simulink model "prob1"  (R2020b)
settings: Solver=VariableStepAuto  StartTime=0.0  StopTime=10.0  RelTol=1e-3
settings Model: Creator=Nitin  LastModifiedBy=Nitin

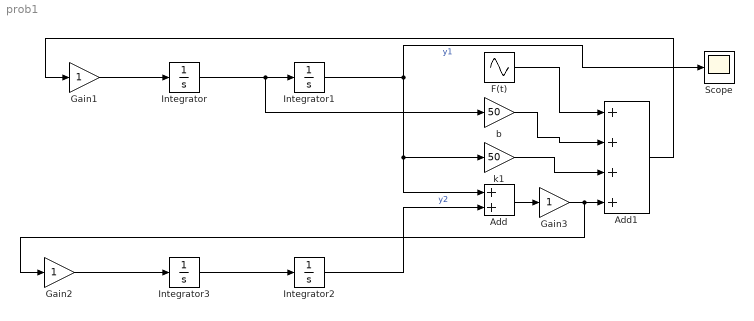
== system prob1 ==
  Add : Sum
  Add1 : Sum  Inputs=++++
  F(t) : Sin  SampleTime=0
  Gain1 : Gain
  Gain2 : Gain
  Gain3 : Gain
  Integrator{,1..3} (4 alike) : Integrator
  Scope : Scope
  b : Gain  Gain=50
  k1 : Gain  Gain=50
  wires:
  k1/1 -> Add1/3
  F(t)/1 -> Add1/1
  Integrator1/1 -> Add/1, k1/1, Scope/1  "y1"
  Add/1 -> Gain3/1
  Gain1/1 -> Integrator/1
  Integrator3/1 -> Integrator2/1
  Integrator/1 -> b/1, Integrator1/1
  Gain2/1 -> Integrator3/1
  Integrator2/1 -> Add/2  "y2"
  Gain3/1 -> Gain2/1, Add1/4
  b/1 -> Add1/2
  Add1/1 -> Gain1/1
